simulink library "CM475A_TSG31CfgAndUse_ModelLibrary_Rev001"  (Simulink 8.2)
settings: Solver=ode45  StartTime=0.0  StopTime=10.0  RelTol=1e-3
values from neighbouring files (symbols this model uses):
  ELECGLBPRM_PWMTMRPERDIVS_CNTPERNANOSEC_U13P19 = DataDict.Constant    [CM475A_TSG31CfgAndUse_DataDict.m]
settings Model: Creator=nz3zln  LastModifiedBy=nz3zln

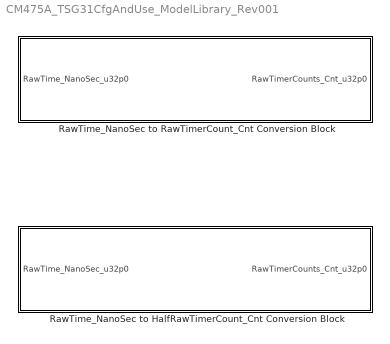
== system CM475A_TSG31CfgAndUse_ModelLibrary_Rev001 ==
  RawTime_NanoSec to HalfRawTimerCount_Cnt Conversion Block : Subsystem  TreatAsAtomicUnit=on
  RawTime_NanoSec to RawTimerCount_Cnt Conversion Block : Subsystem  TreatAsAtomicUnit=on

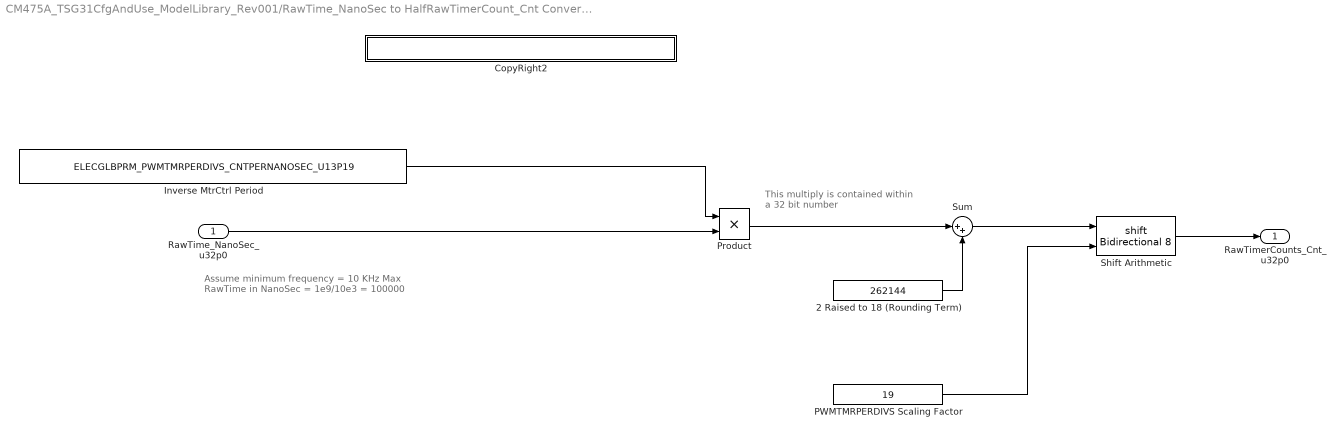
== system CM475A_TSG31CfgAndUse_ModelLibrary_Rev001/RawTime_NanoSec to HalfRawTimerCount_Cnt Conversion Block ==
  note: Assume minimum frequency = 10 KHz
      | Max RawTime in NanoSec = 1e9/10e3 = 100000
  note: This multiply is contained within
      | a 32 bit number
  RawTime_NanoSec_u32p0 : Inport  OutDataTypeStr=uint32
  2 Raised to 18 (Rounding Term) : Constant  Value=262144  OutDataTypeStr=uint32
  CopyRight2 : Subsystem  Description=|  mask(Copyright Information){none=on}
      | Copyright info block.                                               
      |                                                                     
      | Place copyright information at the top of every subsystem in design.
      mask prompts: none "No parameters"
      mask help: Place copyright information at the top of every subsystem in design.
      mask Display:
      | NxtrConf = 'Nxtr Confidential';
      | 
      | sys = bdroot; %handle for the current model ("system")
      | first = get_param(sys,'Created');
      | first = first(end-3:end);  %year is last four digits
      | 
      | last = get_param(sys,'LastModifiedDate');
      | if isempty(last)
      |     last = datestr(now,'yyyy');
      | else
      |     last = last(end-3:end);
      | end
      | 
      | if strcmp(first,last)
      |     fprintf('%s -- Copyright %s Nxtr',NxtrConf,first)
      | else
      |     fprintf('%s -- %s%s- %s Nxtr',NxtrConf,char(169),first,last)
      | end
  Inverse MtrCtrl Period : Constant  Value=ELECGLBPRM_PWMTMRPERDIVS_CNTPERNANOSEC_U13P19  OutDataTypeStr=uint32
  PWMTMRPERDIVS Scaling Factor : Constant  Value=19  OutDataTypeStr=int32
  Product : Product  OutDataTypeStr=uint32
  Shift Arithmetic : ArithShift  BitShiftNumberSource=Input port  BitShiftNumber=8
      settings: InputPortMap=u0,p1
  Sum : Sum  Inputs=|++
  RawTimerCounts_Cnt_u32p0 : Outport
  wires:
  Inverse MtrCtrl Period/1 -> Product/1
  Product/1 -> Sum/1
  RawTime_NanoSec_u32p0/1 -> Product/2
  2 Raised to 18 (Rounding Term)/1 -> Sum/2
  Sum/1 -> Shift Arithmetic/1
  PWMTMRPERDIVS Scaling Factor/1 -> Shift Arithmetic/2
  Shift Arithmetic/1 -> RawTimerCounts_Cnt_u32p0/1

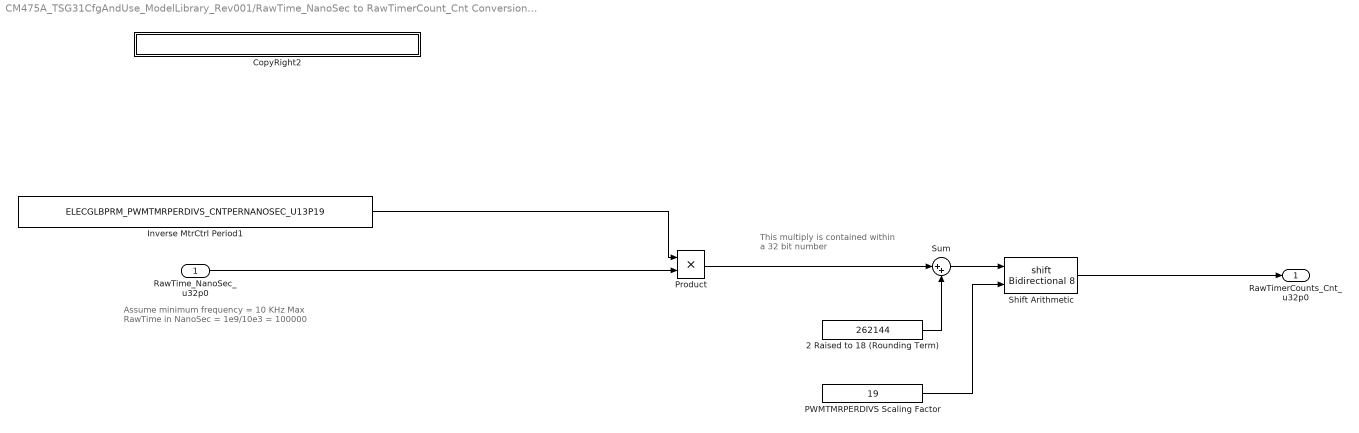
== system CM475A_TSG31CfgAndUse_ModelLibrary_Rev001/RawTime_NanoSec to RawTimerCount_Cnt Conversion Block ==
  note: This multiply is contained within
      | a 32 bit number
  note: Assume minimum frequency = 10 KHz
      | Max RawTime in NanoSec = 1e9/10e3 = 100000
  RawTime_NanoSec_u32p0 : Inport  OutDataTypeStr=uint32
  2 Raised to 18 (Rounding Term) : Constant  Value=262144  OutDataTypeStr=uint32
  CopyRight2 : Subsystem  Description=|  mask(Copyright Information){none=on}
      | Copyright info block.                                               
      |                                                                     
      | Place copyright information at the top of every subsystem in design.
      mask prompts: none "No parameters"
      mask help: Place copyright information at the top of every subsystem in design.
      mask Display:
      | NxtrConf = 'Nxtr Confidential';
      | 
      | sys = bdroot; %handle for the current model ("system")
      | first = get_param(sys,'Created');
      | first = first(end-3:end);  %year is last four digits
      | 
      | last = get_param(sys,'LastModifiedDate');
      | if isempty(last)
      |     last = datestr(now,'yyyy');
      | else
      |     last = last(end-3:end);
      | end
      | 
      | if strcmp(first,last)
      |     fprintf('%s -- Copyright %s Nxtr',NxtrConf,first)
      | else
      |     fprintf('%s -- %s%s- %s Nxtr',NxtrConf,char(169),first,last)
      | end
  Inverse MtrCtrl Period1 : Constant  Value=ELECGLBPRM_PWMTMRPERDIVS_CNTPERNANOSEC_U13P19  OutDataTypeStr=uint32
  PWMTMRPERDIVS Scaling Factor : Constant  Value=19  OutDataTypeStr=int32
  Product : Product  OutDataTypeStr=uint32
  Shift Arithmetic : ArithShift  BitShiftNumberSource=Input port  BitShiftNumber=8
      settings: InputPortMap=u0,p1
  Sum : Sum  Inputs=|++
  RawTimerCounts_Cnt_u32p0 : Outport
  wires:
  RawTime_NanoSec_u32p0/1 -> Product/2
  Product/1 -> Sum/1
  PWMTMRPERDIVS Scaling Factor/1 -> Shift Arithmetic/2
  2 Raised to 18 (Rounding Term)/1 -> Sum/2
  Sum/1 -> Shift Arithmetic/1
  Shift Arithmetic/1 -> RawTimerCounts_Cnt_u32p0/1
  Inverse MtrCtrl Period1/1 -> Product/1

== system CM475A_TSG31CfgAndUse_ModelLibrary_Rev001/RawTime_NanoSec to HalfRawTimerCount_Cnt Conversion Block/CopyRight2 ==

== system CM475A_TSG31CfgAndUse_ModelLibrary_Rev001/RawTime_NanoSec to RawTimerCount_Cnt Conversion Block/CopyRight2 ==
